simulink library "aerolibanim"  (Simulink 5.0)
settings Model: Creator=sgage  LastModifiedBy=sgage  ExtModeAutoUpdateStatusClock=off

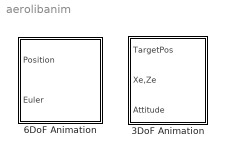
== system aerolibanim ==
  3DoF Animation : Subsystem  mask(3DoF_Animation){u1=[0 5000 -2000 2000 -5050 -3050], u2=0.05, u3=1.0, u5=Fixed position, u6=[2000 500 -3150], u7=10, u8=on}
      mask prompts: u1 "Axes limits [xmin xmax ymin ymax zmin zmax]:"; u2 "Time interval between updates:"; u3 "Size of craft displayed:"; u5 "Enter view:"; u6 "Position of camera [xc yc zc]:"; u7 "View angle:"; u8 "Enable animation"
      mask help:
      | Create a 3-D animated view of a three-degrees-of-freedom craft and its target, where X and Z target position (TargetPos), X and Z craft position (Xe,Ze), and craft attitude are inputs.
      |
      | Display parameters are in the same units of length as the input parameters.
      mask init:
      | Config.axes = u1;
      | Config.update = u2;
      | Config.craft = u3;
      | Config.camera_view = u5;
      | Config.camera_pos = u6;
      | Config.view = u7;
      | Config.Animenable = u8;
      | [xp yp] = aeroimage('anim');
      mask Help: web(asbhelp('3dofanimation'));
      mask StyleString: edit,edit,edit,popup(Fixed position|Cockpit|Fly alongside),edit,edit,checkbox
      mask Display:
      | port_label('input',1,'x_{t},z_{t}','texmode','on');
      | port_label('input',2,'x_e,z_e','texmode','on');
      | port_label('input',3,'\theta','texmode','on');
      | patch(xp,yp)
  6DoF Animation : Subsystem  mask(6DoF_Animation){u1=[0 4000 -2000 2000 -5000 -3000], u2=0.1, u3=1.0, u4=[4000 0 -5000], u5=Fixed position, u6=[2000 500 -3150], u7=10, u8=on}
      mask prompts: u1 "Axes limits [xmin xmax ymin ymax zmin zmax]:"; u2 "Time interval between updates:"; u3 "Size of craft displayed:"; u4 "Static object position [xp yp zp]:"; u5 "Enter view:"; u6 "Position of camera [xc yc zc]:"; u7 "View angle:"; u8 "Enable animation"
      mask help:
      | Create a 3-D animated view of a six-degrees-of-freedom craft, where X, Y, and Z craft position (Position) and craft Euler angles (Euler) are inputs.
      |
      | Display parameters are in the same units of length as the input parameters.
      mask init:
      | Config.axes = u1;
      | Config.update = u2;
      | Config.craft = u3;
      | Config.target = u4;
      | Config.camera_view = u5;
      | Config.camera_pos = u6;
      | Config.view = u7;
      | Config.Animenable = u8;
      | [xp yp] = aeroimage('anim');
      mask Help: web(asbhelp('6dofanimation'));
      mask StyleString: edit,edit,edit,edit,popup(Fixed position|Cockpit|Fly alongside),edit,edit,checkbox
      mask Display:
      | port_label('input',1,'x_e','texmode','on');
      | port_label('input',2,'\phi \theta \psi','texmode','on');
      | patch(xp,yp)

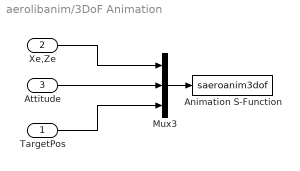
== system aerolibanim/3DoF Animation ==
  TargetPos : Inport
  Xe,Ze : Inport  Port=2
  Attitude : Inport  Port=3
  Animation S-Function : S-Function  FunctionName=saeroanim3dof  Parameters=Config
  Mux3 : Mux  Inputs=3
  wires:
  Xe,Ze/1 -> Mux3/1
  Attitude/1 -> Mux3/2
  TargetPos/1 -> Mux3/3
  Mux3/1 -> Animation S-Function/1

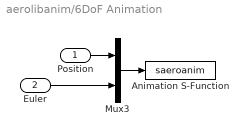
== system aerolibanim/6DoF Animation ==
  Position : Inport
  Euler : Inport  Port=2
  Animation S-Function : S-Function  FunctionName=saeroanim  Parameters=Config
  Mux3 : Mux  Inputs=2
  wires:
  Mux3/1 -> Animation S-Function/1
  Position/1 -> Mux3/1
  Euler/1 -> Mux3/2
